simulink model "chap11_5sim"  (Simulink 6.3)
settings: Solver=ode45  StartTime=0  StopTime=5  RelTol=1e-3
values from neighbouring files (symbols this model uses):
  bc = 30.0    (= 30)    [chap11_4int.m]    (also in chap11_5int.m = 3)
  bl = 8.0    (= 8)    [chap11_5int.m]
  bm = 0.010    (= 0.01)    [chap11_5int.m]
  Ce = 1.2    [chap11_2.m]    (also in chap11_3plant.m; chap11_4int.m = 0.001; chap11_5int.m = 0.001)
  Fc = 0.28    [chap11_1plant.m]    (also in chap11_2plant.m = 15; chap11_3plant.m = 15; chap11_4int.m = 100; chap11_5int.m = 10)
  Jl = 0.15    [chap11_5int.m]
  Jm = 0.005    [chap11_5int.m]
  kd = 6    [chap11_4int.m]    (also in chap11_5int.m; chap11_6int.m)
  kdd = 1.5    [chap11_4int.m]    (also in chap11_5int.m = 50)
  ki = 0.001    [chap11_4int.m]    (also in chap11_5int.m)
  kii = 0.1    [chap11_4int.m]    (also in chap11_5int.m = 1)
  kl = 5.0    (= 5)    [chap11_5int.m]
  km = 1.0    (= 1)    [chap11_4int.m]    (also in chap11_5int.m = 10)
  kpp = 150    [chap11_4int.m]    (also in chap11_5int.m = 100)
  ku = 11    [chap11_4int.m]    (also in chap11_5int.m)
  kv = 2.0    (= 2)    [chap11_2plant.m]    (also in chap11_3plant.m; chap11_4int.m; chap11_5int.m; chap11_6int.m)
  L = 0.001    [chap11_4int.m]    (also in chap11_5int.m)
  R = 7.77    [chap11_2.m]    (also in chap11_3plant.m; chap11_4int.m = 1; chap11_5int.m = 1)
undefined symbols (not defined in the file or in its folder): sgn
libraries: simulink_extras x1
settings Model: LastModifiedBy=Administrator  ExtModeTrigMode=oneshot  ExtModeArmWhenConnect=off  StrictBusMsg=None
settings DataIOCC: LimitDataPoints=off
settings OptimizationCC: BlockReduction=off  BooleanDataType=off
settings DebuggingCC: SolverPrmCheckMsg=none
settings HardwareCC: TargetUnknown=on

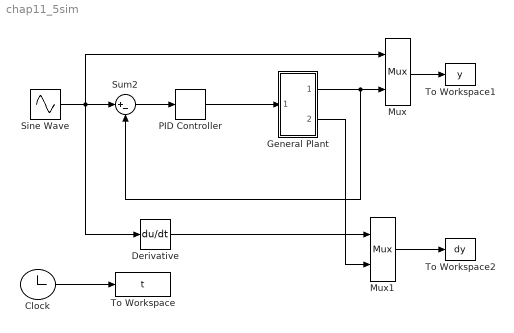
== system chap11_5sim ==
  Clock : Clock
      settings: Decimation=10
  Derivative : Derivative
  General Plant : Subsystem
  Mux : Mux  Inputs=2
  Mux1 : Mux  Inputs=2
  PID Controller : simulink_extras/Additional Linear/PID Controller  P=kpp  I=kii  D=kdd
  Sine Wave : Sin  Frequency=2*pi  SampleTime=0
  Sum2 : Sum  Inputs=|+-  SaturateOnIntegerOverflow=on  InputSameDT=on
  To Workspace : ToWorkspace  VariableName=t  SampleTime=-1  SaveFormat=Array
  To Workspace1 : ToWorkspace  VariableName=y  SampleTime=-1  SaveFormat=Array
  To Workspace2 : ToWorkspace  VariableName=dy  SampleTime=-1  SaveFormat=Array
  wires:
  Mux/1 -> To Workspace1/1
  Mux1/1 -> To Workspace2/1
  General Plant/1(Out1) -> Mux/2, Sum2/2
  Sum2/1 -> PID Controller/1
  Sine Wave/1 -> Mux/1, Sum2/1, Derivative/1
  PID Controller/1 -> General Plant/1(In1)
  Clock/1 -> To Workspace/1
  Derivative/1 -> Mux1/1
  General Plant/2(Out2) -> Mux1/2

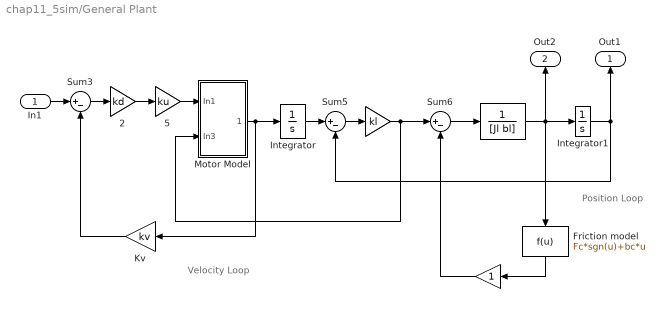
== system chap11_5sim/General Plant ==
  note: Velocity Loop
  note: Position Loop
  In1 : Inport
  " " : Gain  Gain=kl  SaturateOnIntegerOverflow=on
  "   " : Gain  Orientation=left  SaturateOnIntegerOverflow=on
  "    " : TransferFcn  Denominator=[Jl bl]
  " 2" : Gain  Gain=kd  SaturateOnIntegerOverflow=on
  " 5" : Gain  Gain=ku  SaturateOnIntegerOverflow=on
  Friction model : Fcn  Orientation=down  Expr=Fc*sgn(u)+bc*u
  Integrator : Integrator
  Integrator1 : Integrator
  Kv : Gain  Orientation=left  Gain=kv  SaturateOnIntegerOverflow=on
  Motor Model : Subsystem
  Sum3 : Sum  Inputs=|+-  SaturateOnIntegerOverflow=on  InputSameDT=on
  Sum5 : Sum  Inputs=|+-  SaturateOnIntegerOverflow=on  InputSameDT=on
  Sum6 : Sum  Inputs=|+-  SaturateOnIntegerOverflow=on  InputSameDT=on
  Out1 : Outport  Orientation=up
  Out2 : Outport  Orientation=up  Port=2
  wires:
  Kv/1 -> Sum3/2
  Motor Model/1(Out1) -> Integrator/1, Kv/1
  In1/1 -> Sum3/1
  Sum3/1 -> " 2"/1
  " 2"/1 -> " 5"/1
  " 5"/1 -> Motor Model/1(In1)
  Sum5/1 -> " "/1
  Integrator/1 -> Sum5/1
  Integrator1/1 -> Sum5/2, Out1/1
  Sum6/1 -> "    "/1
  " "/1 -> Sum6/1, Motor Model/2(In3)
  "    "/1 -> Friction model/1, Integrator1/1, Out2/1
  Friction model/1 -> "   "/1
  "   "/1 -> Sum6/2

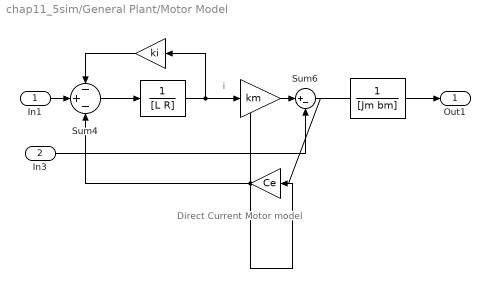
== system chap11_5sim/General Plant/Motor Model ==
  note: i
  note: Direct Current Motor model
  In1 : Inport
  In3 : Inport  Port=2
  "    " : Gain  Orientation=left  Gain=Ce  SaturateOnIntegerOverflow=on
  "      " : Gain  Orientation=left  Gain=ki  SaturateOnIntegerOverflow=on
  "  " : Gain  Gain=km  SaturateOnIntegerOverflow=on
  "   " : TransferFcn  Denominator=[L R]
  "    " : TransferFcn  Denominator=[Jm bm]
  Sum4 : Sum  Inputs=-+-  InputSameDT=on
  Sum6 : Sum  Inputs=|+-  SaturateOnIntegerOverflow=on  InputSameDT=on
  Out1 : Outport
  wires:
  "    "/1 -> "    "/1, Out1/1
  Sum4/1 -> "   "/1
  "   "/1 -> "      "/1, "  "/1
  "      "/1 -> Sum4/1
  In1/1 -> Sum4/2
  "  "/1 -> Sum6/1
  In3/1 -> Sum6/2
  "    "/1 -> Sum4/3
  Sum6/1 -> "    "/1
